simulink model "STBC1"  (Simulink 6.5)
settings: Solver=ode45  StartTime=0.0  StopTime=inf  RelTol=1e-3
undefined symbols (not defined in the file): magnitude
libraries: commsequence2 x8, commchan3 x3, commdigbbndpm3 x2, dspstat3 x2, dspmtrx3 x2, commsink2 x1, commrandsrc2 x1
settings Model: Creator=koko  LastModifiedBy=koko

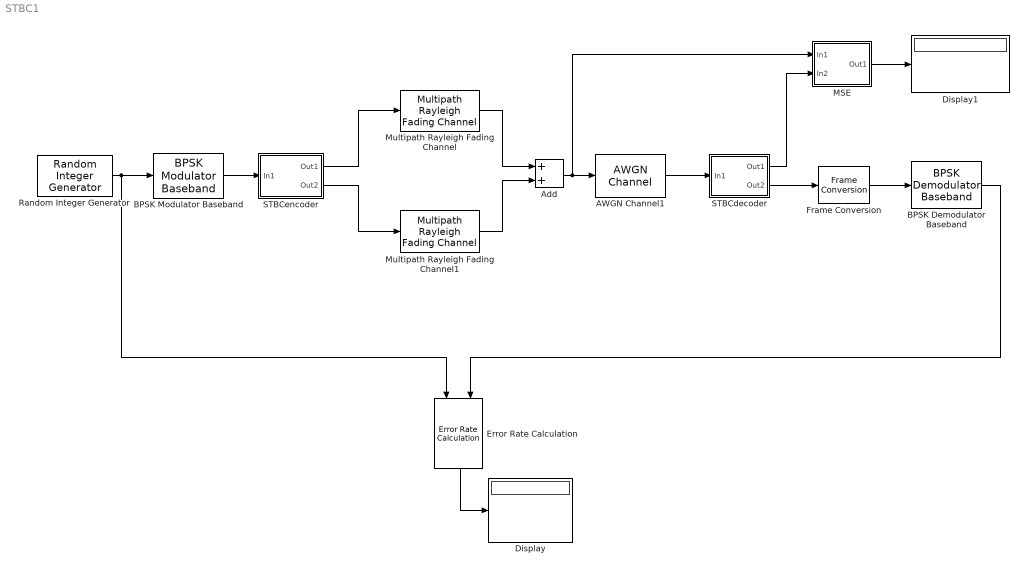
== system STBC1 ==
  AWGN Channel1 : commchan3/AWGN Channel  SystemSampleTime=-1  seed=18293  noiseMode="Signal to noise ratio  (Eb/No)"  EbNodB=12  EsNodB=10  SNRdB=10  bitsPerSym=1  Ps=1  Tsym=0.0000005  variance=1
  Add : Sum  OutScaling=2^-10
  BPSK Demodulator Baseband : commdigbbndpm3/BPSK Demodulator Baseband  DialogController=commDDGCreate  DialogControllerArgs=DataTag0  Ph=0  DecType=Hard decision  VarSource=Dialog  Variance=1  outDtype=double
  BPSK Modulator Baseband : commdigbbndpm3/BPSK Modulator Baseband  SystemSampleTime=-1  Ph=0  outDtype=double  outWordLen=16  outUDDataType=sfix(16)  outFracLenMode=Best precision  outFracLen=15
  Display : Display
  Display1 : Display
  Error Rate Calculation : commsink2/Error Rate Calculation  Orientation=down  N=0  st_delay=0  cp_mode=Entire frame  subframe=[]  PMode=Port  WsName=ErrorVec  RsMode2=off  stop=on  numErr=1000000  maxBits=5e5
  Frame Conversion : FrameConversion
  MSE : Subsystem
  Multipath Rayleigh Fading Channel : commchan3/Multipath Rayleigh Fading Channel  SystemSampleTime=-1  maxDopplerShift=40  pathDelays=[0]  avgPathGaindB=[0]  normalizePathGains=on  seed=73117  enableProbe=0  openVisAtStart=off  outPathGains=off  outDelay=off
  Multipath Rayleigh Fading Channel1 : commchan3/Multipath Rayleigh Fading Channel  SystemSampleTime=-1  maxDopplerShift=40  pathDelays=[0]  avgPathGaindB=[0]  normalizePathGains=on  seed=17893  enableProbe=0  openVisAtStart=off  outPathGains=off  outDelay=off
  Random Integer Generator : commrandsrc2/Random Integer Generator  SystemSampleTime=-1  mul=2  seed=871234  Ts=1e-6  frameBased=on  sampPerFrame=2  orient=off  outDataType=double
  STBCdecoder : Subsystem
  STBCencoder : Subsystem
  wires:
  BPSK Modulator Baseband/1 -> STBCencoder/1(In1)
  STBCencoder/1(Out1) -> Multipath Rayleigh Fading Channel/1
  STBCencoder/2(Out2) -> Multipath Rayleigh Fading Channel1/1
  Error Rate Calculation/1 -> Display/1
  Random Integer Generator/1 -> BPSK Modulator Baseband/1, Error Rate Calculation/1
  Multipath Rayleigh Fading Channel/1 -> Add/1
  Multipath Rayleigh Fading Channel1/1 -> Add/2
  Add/1 -> AWGN Channel1/1, MSE/1(In1)
  AWGN Channel1/1 -> STBCdecoder/1(In1)
  BPSK Demodulator Baseband/1 -> Error Rate Calculation/2
  Frame Conversion/1 -> BPSK Demodulator Baseband/1
  STBCdecoder/2(Out2) -> Frame Conversion/1
  STBCdecoder/1(Out1) -> MSE/2(In2)
  MSE/1(Out1) -> Display1/1

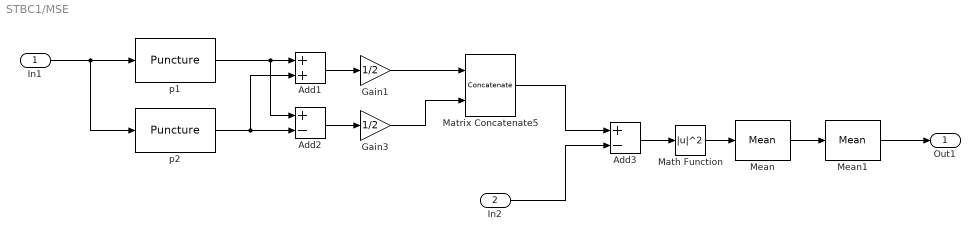
== system STBC1/MSE ==
  In1 : Inport
  In2 : Inport  Port=2
  Add1 : Sum  OutScaling=2^-10
  Add2 : Sum  Inputs=+-  OutScaling=2^-10
  Add3 : Sum  Inputs=+-  OutScaling=2^-10
  Gain1 : Gain  Gain=1/2
  Gain3 : Gain  Gain=1/2
  Math Function : Math  Operator=magnitude^2  SaturateOnIntegerOverflow=on
  Matrix Concatenate5 : Concatenate  Mode=Vertical matrix concatenation
  Mean : dspstat3/Mean  DialogController=dspDDGCreate  DialogControllerArgs=DataTag1  run=on  reset_popup=None  roundingMode=Floor  overflowMode=off
  Mean1 : dspstat3/Mean  DialogController=dspDDGCreate  DialogControllerArgs=DataTag2  run=off  reset_popup=None  roundingMode=Floor  overflowMode=off
  p1 : commsequence2/Puncture  punctureVector=[1 0 0 0].'
  p2 : commsequence2/Puncture  punctureVector=[0 1 0 0].'
  Out1 : Outport
  wires:
  p1/1 -> Add1/1, Add2/1
  p2/1 -> Add2/2, Add1/2
  Add1/1 -> Gain1/1
  Add2/1 -> Gain3/1
  In1/1 -> p1/1, p2/1
  Gain3/1 -> Matrix Concatenate5/2
  Gain1/1 -> Matrix Concatenate5/1
  Matrix Concatenate5/1 -> Add3/1
  Mean/1 -> Mean1/1
  In2/1 -> Add3/2
  Add3/1 -> Math Function/1
  Math Function/1 -> Mean/1
  Mean1/1 -> Out1/1

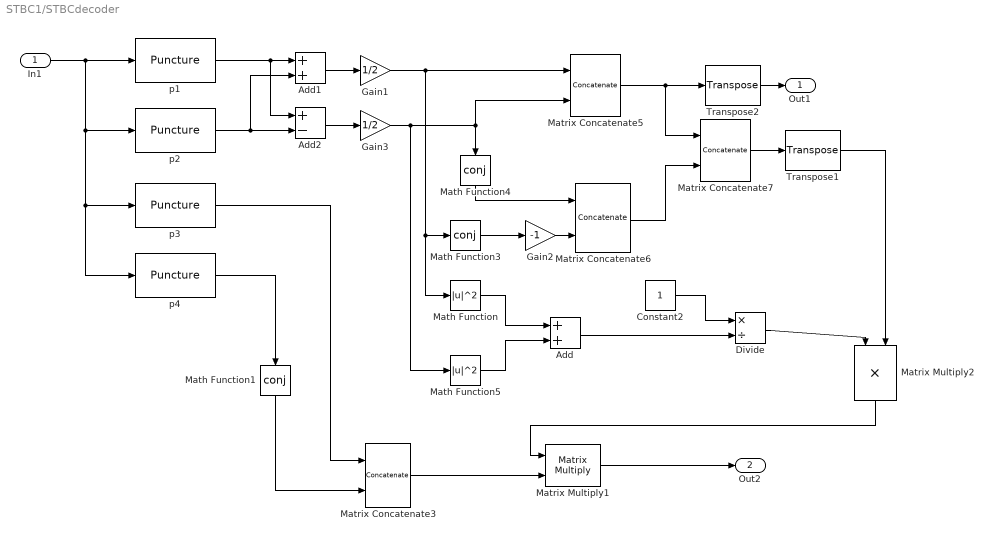
== system STBC1/STBCdecoder ==
  In1 : Inport
  Add : Sum  OutScaling=2^-10
  Add1 : Sum  OutScaling=2^-10
  Add2 : Sum  Inputs=+-  OutScaling=2^-10
  Constant2 : Constant  Value=1  OutDataType=sfix(16)  ConRadixGroup=Use specified scaling  OutScaling=2^0  SampleTime=inf  FramePeriod=inf
  Divide : Product  Inputs=*/  OutScaling=2^-10
  Gain1 : Gain  Gain=1/2
  Gain2 : Gain  Gain=-1
  Gain3 : Gain  Gain=1/2
  Math Function : Math  Operator=magnitude^2  SaturateOnIntegerOverflow=on
  Math Function1 : Math  Orientation=down  Operator=conj  SaturateOnIntegerOverflow=on
  Math Function3 : Math  Operator=conj  SaturateOnIntegerOverflow=on
  Math Function4 : Math  Orientation=down  Operator=conj  SaturateOnIntegerOverflow=on
  Math Function5 : Math  Operator=magnitude^2  SaturateOnIntegerOverflow=on
  Matrix Concatenate3 : Concatenate  Mode=Vertical matrix concatenation
  Matrix Concatenate5 : Concatenate  Mode=Horizontal matrix concatenation
  Matrix Concatenate6 : Concatenate  Mode=Horizontal matrix concatenation
  Matrix Concatenate7 : Concatenate  Mode=Vertical matrix concatenation
  Matrix Multiply1 : Product  Multiplication=Matrix(*)
  Matrix Multiply2 : Product  Orientation=down
  Transpose1 : dspmtrx3/Transpose  SystemSampleTime=-1  Hermitian=on  overflowFlag=off
  Transpose2 : dspmtrx3/Transpose  SystemSampleTime=-1  Hermitian=off  overflowFlag=off
  p1 : commsequence2/Puncture  punctureVector=[1 0 0 0].'
  p2 : commsequence2/Puncture  punctureVector=[0 1 0 0].'
  p3 : commsequence2/Puncture  punctureVector=[0 0 1 0].'
  p4 : commsequence2/Puncture  punctureVector=[0 0 0 1].'
  Out1 : Outport
  Out2 : Outport  Port=2
  wires:
  p4/1 -> Math Function1/1
  p3/1 -> Matrix Concatenate3/1
  Matrix Concatenate5/1 -> Matrix Concatenate7/1, Transpose2/1
  Matrix Concatenate6/1 -> Matrix Concatenate7/2
  Matrix Concatenate7/1 -> Transpose1/1
  Gain2/1 -> Matrix Concatenate6/2
  Math Function4/1 -> Matrix Concatenate6/1
  Math Function3/1 -> Gain2/1
  Matrix Concatenate3/1 -> Matrix Multiply1/2
  Transpose1/1 -> Matrix Multiply2/2
  Matrix Multiply2/1 -> Matrix Multiply1/1
  Matrix Multiply1/1 -> Out2/1
  p1/1 -> Add1/1, Add2/1
  p2/1 -> Add2/2, Add1/2
  Add1/1 -> Gain1/1
  Add2/1 -> Gain3/1
  Divide/1 -> Matrix Multiply2/1
  Constant2/1 -> Divide/1
  Add/1 -> Divide/2
  Math Function5/1 -> Add/2
  Gain1/1 -> Matrix Concatenate5/1, Math Function3/1, Math Function/1
  Math Function/1 -> Add/1
  Math Function1/1 -> Matrix Concatenate3/2
  Gain3/1 -> Math Function4/1, Matrix Concatenate5/2, Math Function5/1
  In1/1 -> p1/1, p2/1, p3/1, p4/1
  Transpose2/1 -> Out1/1

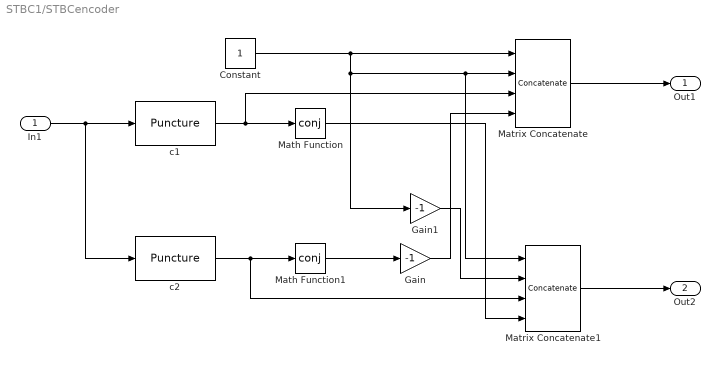
== system STBC1/STBCencoder ==
  In1 : Inport
  Constant : Constant  Value=1  OutDataType=sfix(16)  ConRadixGroup=Use specified scaling  OutScaling=2^0  SampleTime=inf  FramePeriod=inf
  Gain : Gain  Gain=-1
  Gain1 : Gain  Gain=-1
  Math Function : Math  Operator=conj  SaturateOnIntegerOverflow=on
  Math Function1 : Math  Operator=conj  SaturateOnIntegerOverflow=on
  Matrix Concatenate : Concatenate  NumInputs=4  Mode=Vertical matrix concatenation
  Matrix Concatenate1 : Concatenate  NumInputs=4  Mode=Vertical matrix concatenation
  c1 : commsequence2/Puncture  punctureVector=[1 0].'
  c2 : commsequence2/Puncture  punctureVector=[0 1].'
  Out1 : Outport
  Out2 : Outport  Port=2
  wires:
  In1/1 -> c1/1, c2/1
  c1/1 -> Math Function/1, Matrix Concatenate/3
  c2/1 -> Math Function1/1, Matrix Concatenate1/3
  Math Function1/1 -> Gain/1
  Gain/1 -> Matrix Concatenate/4
  Matrix Concatenate/1 -> Out1/1
  Math Function/1 -> Matrix Concatenate1/4
  Matrix Concatenate1/1 -> Out2/1
  Gain1/1 -> Matrix Concatenate1/2
  Constant/1 -> Matrix Concatenate/1, Matrix Concatenate/2, Matrix Concatenate1/1, Gain1/1
